simulink model "stm32_hwi_gettingstarted"  (R2024b)
settings: Solver=FixedStepAuto  StartTime=0.0  StopTime=inf  RelTol=1e-3  EnableMultiTasking=on
libraries: stm32f4xxblockslib x2, simulink x1
settings Model: STM32="{\"HardwareInterrupt\":{\"ID\":\"stm32_hwi_gettingstarted:47\"},\"DigitalPortWrite\":{\"ID\":\"stm32_hwi_gettingstarted:48\"}}"  Creator=The MathWorks, Inc.  LastModifiedBy=camer
settings SolverCC: AutoInsertRateTranBlk=on
settings OptimizationCC: EnhancedBackFolding=on  PassReuseOutputArgsAs=Individual arguments  ZeroExternalMemoryAtStartup=off  ZeroInternalMemoryAtStartup=off  MaxStackSize=512  OptimizeBlockOrder=speed  DifferentSizesBufferReuse=on  OptimizationCustomize=off  EfficientTunableParamExpr=on
settings DebuggingCC: ParameterTunabilityLossMsg=error  UnconnectedInputMsg=warning  UnconnectedOutputMsg=warning  UnconnectedLineMsg=warning  SubsystemReferenceDiagnosticForUnitTest=warning
settings HardwareCC: ProdBitPerPointer=32  ProdBitPerSizeT=32  ProdBitPerPtrDiffT=32  ProdLargestAtomicInteger=Long  ProdLargestAtomicFloat=Double  ProdWordSize=32  ProdLongLongMode=on  ProdHWDeviceType=ARM Compatible->ARM Cortex
settings ModelReferenceCC: EnableRefExpFcnMdlSchedulingChecks=on
settings SFSimCC: MATLABDynamicMemAlloc=off
settings RTWCC: Description=Embedded Coder  SystemTargetFile=ert.tlc  HardwareBoard=STM32F4xx Based  TemplateMakefile=ert_default_tmf  Toolchain=GNU Tools for ARM Embedded Processors  GPUComputeCapability=3.5  DLArmComputeVersion=19.05
settings CodeAppCC: ForceParamTrailComments=on  IgnoreCustomStorageClasses=off  OperatorAnnotations=on  SimulinkDataObjDesc=on  SFDataObjDesc=on  InsertBlockDesc=on
settings ERTTargetCC: CodeReplacementLibrary=ARM Cortex-M  ExtModeTransport=3  ExtModeStaticAlloc=on  ExtModeStaticAllocSize=8000  ExtModeMexFile=ext_xcp  ExtModeIntrfLevel=Level2 - Open  InlinedParameterPlacement=Hierarchical  DynamicArrayContainerType=coder::array

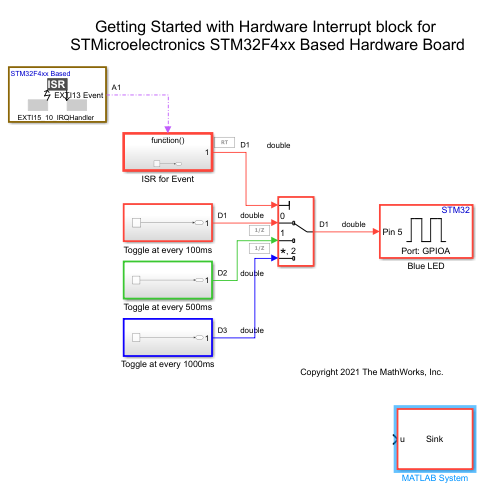
[thumbnail: Simulink's stored preview of the top-level diagram]
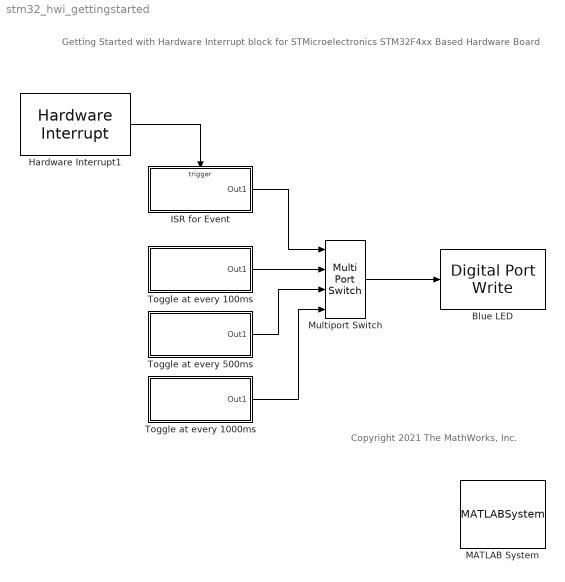
== system stm32_hwi_gettingstarted ==
  note: Getting Started with Hardware Interrupt block for
      | STMicroelectronics STM32F4xx Based Hardware Board
  note: Copyright 2021 The MathWorks, Inc.
  Blue LED : stm32f4xxblockslib/Digital Port Write  PortName=GPIOA  PinNumber=5  ReadOperation=off  IOAsArray=off  EnableSimPort=off  hoistedMaskSrc=ECSoC/ECSimCodegen/Digital Port Write
  Hardware Interrupt1 : stm32f4xxblockslib/Hardware Interrupt  ISRGroup=External interrupts (EXTI)  ISRName=EXTI15_10_IRQHandler  ISRNumber=55  EventsList={ 'off', 'EXTI15 Event', '1'; 'off', 'EXTI14 Event', '2'; 'on', 'EXTI13 Event', '3'; 'off', 'EXTI12 Event', '4'; 'off', 'EXTI11 Event', '5'; 'off', 'EXTI10 Event', '6'; 'off', 'Custom event', '7' }  SelectedEvents={'EXTI13 Event'}  TaskPriority=30  DisablePreemption=off  ClearInterruptFlagsAtEndOfEvent=off  InterruptDefinitionFile=$(TARGET_ROOT)/registry/interrupts/STM32F4xxBased_interrupts.xml  HardwareBoard=STM32F4xx Based  EnableSimPort=off
  ISR for Event : Subsystem  TreatAsAtomicUnit=on
  MATLAB System : MATLABSystem  System=Sink
      mask Type: Sink
      mask Display:
      | disp('Sink');
      | port_label('input',1,'u');
  Multiport Switch : MultiPortSwitch  DataPortOrder=Zero-based contiguous  zeroidx=on  SaturateOnIntegerOverflow=off  InputSameDT=off
  Toggle at every 1000ms : Subsystem
  Toggle at every 100ms : Subsystem
  Toggle at every 500ms : Subsystem
  wires:
  Toggle at every 500ms/1(Out1) -> Multiport Switch/3
  Toggle at every 1000ms/1(Out1) -> Multiport Switch/4
  ISR for Event/1(Out1) -> Multiport Switch/1
  Toggle at every 100ms/1(Out1) -> Multiport Switch/2
  Hardware Interrupt1/1 -> ISR for Event/Trigger
  Multiport Switch/1 -> Blue LED/1

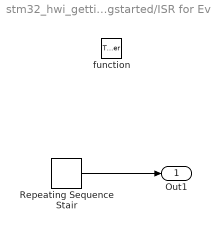
== system stm32_hwi_gettingstarted/ISR for Event ==
  function : TriggerPort  TriggerType=function-call  VariantControl=(inherit)
  Repeating Sequence Stair : simulink/Sources/Repeating Sequence Stair  OutValues=[1 2 0]  tsamp=-1  OutMin=[]  OutMax=[]  OutDataTypeStr=double  OutputDataTypeScalingMode=double  OutDataType=fixdt(0,8)  ConRadixGroup=Best Precision: Vector-wise  OutScaling=2^-12
  Out1 : Outport
  wires:
  Repeating Sequence Stair/1 -> Out1/1

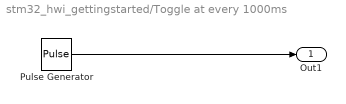
== system stm32_hwi_gettingstarted/Toggle at every 1000ms ==
  Pulse Generator : DiscretePulseGenerator
  Out1 : Outport
  wires:
  Pulse Generator/1 -> Out1/1

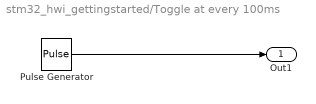
== system stm32_hwi_gettingstarted/Toggle at every 100ms ==
  Pulse Generator : DiscretePulseGenerator  SampleTime=0.1
  Out1 : Outport
  wires:
  Pulse Generator/1 -> Out1/1

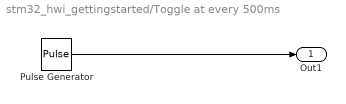
== system stm32_hwi_gettingstarted/Toggle at every 500ms ==
  Pulse Generator : DiscretePulseGenerator  SampleTime=0.5
  Out1 : Outport
  wires:
  Pulse Generator/1 -> Out1/1
